simulink model "grid_tied_Inverter"  (R2013a)
settings: Solver=ode45  SolverMode=SingleTasking  StartTime=0.0  StopTime=5  FixedStep=0.00001  RelTol=1e-3
libraries: powerlib x15, simulink_extras x2, powerlib_extras x2, simulink x1
settings Model: Creator=lang  LastModifiedBy=Yooshaa
settings DataIOCC: SignalLoggingSaveFormat=ModelDataLogs
settings OptimizationCC: BlockReduction=off  BooleanDataType=off  InlineParams=on
settings DebuggingCC: SaveWithParameterizedLinksMsg=none  SignalResolutionControl=TryResolveAllWithWarning  SolverPrmCheckMsg=none  MultiTaskDSMMsg=warning  MultiTaskCondExecSysMsg=none  StrictBusMsg=None
settings HardwareCC: TargetUnknown=on
settings RTWCC: IncludeERTFirstTime=on

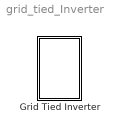
== system grid_tied_Inverter ==
  Grid Tied Inverter : Subsystem  mask{Vdc=1200, Pb=2.3e6, Vp=((690*(2^0.5))/(3^0.5)), Fb=60, Vbase=((690*(2^0.5))/(3^0.5))/(2^.5), Ibase=(2.3e6/3)/(690/(3^0.5)), Grid_Angle_init=pi, Lgrid=0.1098e-3, Fs=1e4, Fsampling=2e4, Kp=1, Ki=2, P_desired_pu=3, Q_desired_pu=0}

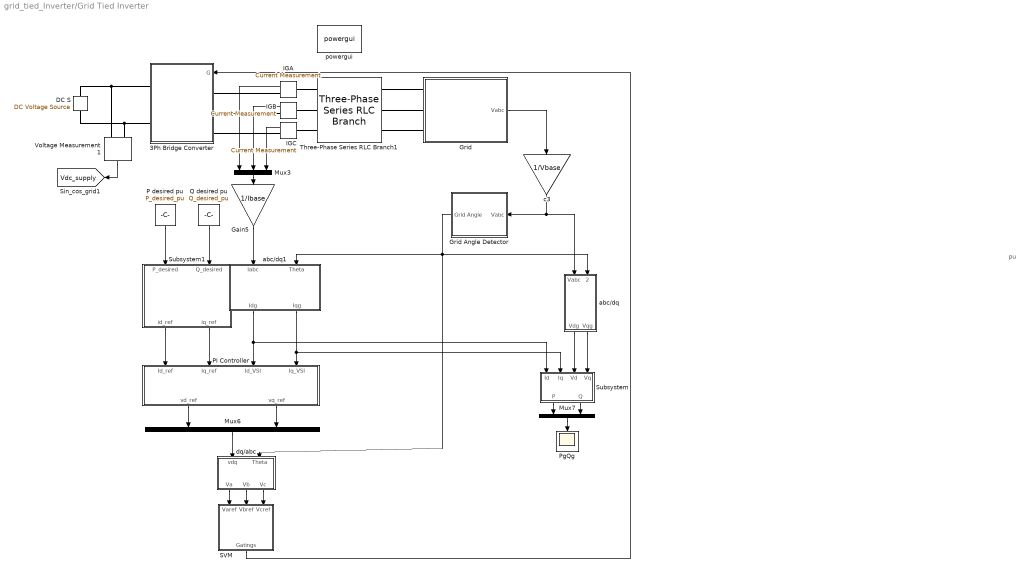
== system grid_tied_Inverter/Grid Tied Inverter ==
  note: pu
  3Ph Bridge Converter : Subsystem
  DC S : powerlib/Electrical Sources/DC Voltage Source  Amplitude=Vdc  Measurements=None
  Gain5 : Gain  Gain=1/Ibase
  Grid : Subsystem
  Grid Angle Detector : Subsystem
  IGA : powerlib/Measurements/Current Measurement  PhasorSimulation=off  OutputType=Complex  PSBequivalent=0
  IGB : powerlib/Measurements/Current Measurement  PhasorSimulation=off  OutputType=Complex  PSBequivalent=0
  IGC : powerlib/Measurements/Current Measurement  PhasorSimulation=off  OutputType=Complex  PSBequivalent=0
  Mux3 : Mux  Inputs=3
  Mux6 : Mux  Inputs=2
  Mux7 : Mux  Inputs=2
  P desired pu : Constant  Value=P_desired_pu
  PI Controller : Subsystem
  PgQg : Scope
      settings: YMin=-2  YMax=6  SaveName=ScopeData7
  Q desired pu : Constant  Value=Q_desired_pu
  SVM : Subsystem
  Subsystem : Subsystem
  Subsystem1 : Subsystem
  Three-Phase Series RLC Branch1 : powerlib/Elements/Three-Phase Series RLC Branch  LConnTagsString=A|B|C  RConnTagsString=A|B|C  BranchType=L  Resistance=1e-6  Inductance=Lgrid  Capacitance=1e-6  Measurements=Branch currents
  Voltage Measurement1 : powerlib/Measurements/Voltage Measurement  PhasorSimulation=off  OutputType=Complex  PSBequivalent=0
  abc/dq : Subsystem
  abc/dq1 : Subsystem
  c3 : Gain  Gain=1/Vbase
  dq/abc : Subsystem
  powergui : powerlib/powergui  Priority=1  SimulationMode=Continuous  SolverType=Tustin  SampleTime=50e-6  frequency=60  SPID=on  DisableSnubberDevices=off  DisableRonSwitches=off  DisableVfSwitches=off  SwTol=0  Interpol=off  DisplayEquations=off  frequencyindice=0  Pbase=100e6  ErrMax=1e-4  Iterations=50  UnitsV=kV  UnitsW=MW  FunctionMessages=off  echomessages=off  HookPort=off  EnableUseOfTLC=off  x0status=blocks  RestoreLinks=warning  ResistiveCurrentMeasurement=off  Frange=[0:2:500]  Ylog=off  Xlog=on  ShowGrid=off  save=off  variable=ZData  ZoomFFT=off  StartTime=0.0  cycles=1  DisplayStyle=1  fundamental=60  FreqAxis=off  MaxFrequency=1000  frequencyindicesteady=1  RmsSteady=1  display=off  Ts=0  methode=off
  tag scope: Vdc_supply=global
  wires:
  Voltage Measurement1/1 -> [Vdc_supply]
  SVM/1(Gatings) -> 3Ph Bridge Converter/1(G)
  dq/abc/2(Vb) -> SVM/2(Vbref)
  Grid/1(Vabc) -> c3/1
  dq/abc/3(Vc) -> SVM/3(Vcref)
  dq/abc/1(Va) -> SVM/1(Varef)
  abc/dq/1(Vdg) -> Subsystem/3(Vd)
  Subsystem1/1(id_ref) -> PI Controller/1(Id_ref)
  abc/dq1/1(Idg) -> PI Controller/3(Id_VSI), Subsystem/1(Id)
  Mux3/1 -> Gain5/1
  PI Controller/2(vq_ref) -> Mux6/2
  IGC/1 -> Mux3/3
  c3/1 -> Grid Angle Detector/1(Vabc), abc/dq/1(Vabc)
  Mux6/1 -> dq/abc/1(vdq)
  Mux7/1 -> PgQg/1
  Subsystem1/2(iq_ref) -> PI Controller/2(Iq_ref)
  Subsystem/2(Q) -> Mux7/2
  IGA/1 -> Mux3/1
  Gain5/1 -> abc/dq1/1(Iabc)
  Subsystem/1(P) -> Mux7/1
  abc/dq1/2(Iqg) -> Subsystem/2(Iq), PI Controller/4(Iq_VSI)
  IGB/1 -> Mux3/2
  Grid Angle Detector/1(Grid Angle) -> dq/abc/2(Theta), abc/dq1/2(Theta), abc/dq/2(Theta)
  PI Controller/1(vd_ref) -> Mux6/1
  abc/dq/2(Vqg) -> Subsystem/4(Vq)
  P desired pu/1 -> Subsystem1/1(P_desired)
  Q desired pu/1 -> Subsystem1/2(Q_desired)
  connections:
  3Ph Bridge Converter/RConn1 -- DC S/RConn1 -- Voltage Measurement1/LConn1
  3Ph Bridge Converter/RConn2 -- DC S/LConn1 -- Voltage Measurement1/LConn2
  IGC/RConn1 -- 3Ph Bridge Converter/LConn3
  Three-Phase Series RLC Branch1/RConn1 -- IGA/LConn1
  Three-Phase Series RLC Branch1/RConn3 -- IGC/LConn1
  3Ph Bridge Converter/LConn1 -- IGA/RConn1
  Three-Phase Series RLC Branch1/RConn2 -- IGB/LConn1
  Grid/LConn1 -- Three-Phase Series RLC Branch1/LConn1
  Grid/LConn2 -- Three-Phase Series RLC Branch1/LConn2
  3Ph Bridge Converter/LConn2 -- IGB/RConn1
  Grid/LConn3 -- Three-Phase Series RLC Branch1/LConn3

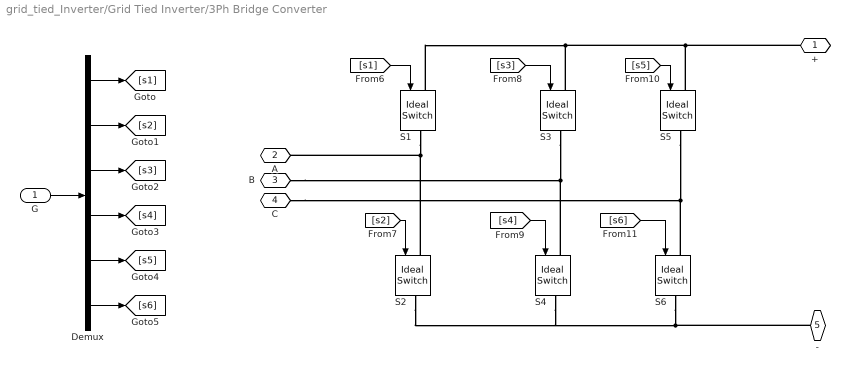
== system grid_tied_Inverter/Grid Tied Inverter/3Ph Bridge Converter ==
  G : Inport
   S{1..6} (6 alike) : powerlib/Power Electronics/Ideal Switch  Ron=0  Lon=0  IC=0  Rs=inf  Cs=inf  Measurements=off
  Demux : Demux  Outputs=6
  + : PMIOPort  Port=1  Side=Right
  A : PMIOPort  Port=2  Side=Left
  B : PMIOPort  Port=3  Side=Left
  C : PMIOPort  Port=4  Side=Left
  - : PMIOPort  Port=5  Side=Right
  wires:
  [s1] -> " S1"/1
  [s5] -> " S5"/1
  Demux/1 -> [s1]
  Demux/2 -> [s2]
  Demux/3 -> [s3]
  Demux/4 -> [s4]
  Demux/5 -> [s5]
  Demux/6 -> [s6]
  G/1 -> Demux/1
  [s2] -> " S2"/1
  [s3] -> " S3"/1
  [s4] -> " S4"/1
  [s6] -> " S6"/1
  connections:
  +/RConn1 -- " S1"/LConn1 -- " S3"/LConn1 -- " S5"/LConn1
  -/RConn1 -- " S2"/RConn1 -- " S4"/RConn1 -- " S6"/RConn1
  " S1"/RConn1 -- " S2"/LConn1 -- A/RConn1
  B/RConn1 -- " S4"/LConn1 -- " S3"/RConn1
  C/RConn1 -- " S6"/LConn1 -- " S5"/RConn1

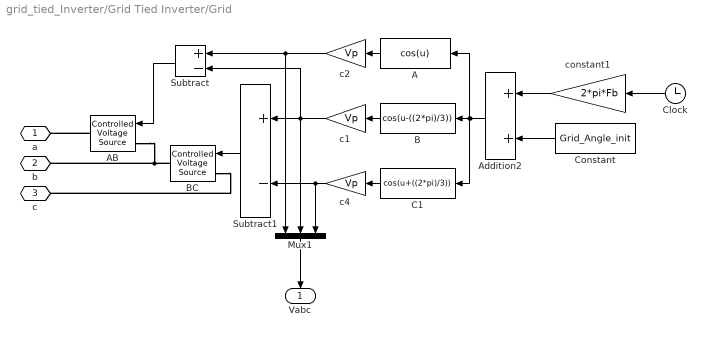
== system grid_tied_Inverter/Grid Tied Inverter/Grid ==
  A : Fcn  Expr=cos(u)
  AB : powerlib/Electrical Sources/Controlled Voltage Source  Initialize=off  Source_Type=AC  Amplitude=0  Phase=0  Frequency=0  Measurements=None
  Addition2 : Sum
  B : Fcn  Expr=cos(u-((2*pi)/3))
  BC : powerlib/Electrical Sources/Controlled Voltage Source  Initialize=off  Source_Type=AC  Amplitude=0  Phase=0  Frequency=0  Measurements=None
  C1 : Fcn  Expr=cos(u+((2*pi)/3))
  Clock : Clock
  Constant : Constant  Value=Grid_Angle_init
  Mux1 : Mux  Inputs=3
  Subtract : Sum  Inputs=+-
  Subtract1 : Sum  Inputs=+-
  c1 : Gain  Gain=Vp
  c2 : Gain  Gain=Vp
  c4 : Gain  Gain=Vp
  constant1 : Gain  Gain=2*pi*Fb
  a : PMIOPort  Port=1  Side=Left
  b : PMIOPort  Port=2  Side=Left
  c : PMIOPort  Port=3  Side=Left
  Vabc : Outport
  wires:
  c4/1 -> Subtract1/2, Mux1/3
  constant1/1 -> Addition2/1
  c1/1 -> Subtract1/1, Mux1/2, Subtract/2
  Addition2/1 -> C1/1, A/1, B/1
  Constant/1 -> Addition2/2
  B/1 -> c1/1
  C1/1 -> c4/1
  Clock/1 -> constant1/1
  c2/1 -> Subtract/1, Mux1/1
  A/1 -> c2/1
  Subtract1/1 -> BC/1
  Mux1/1 -> Vabc/1
  Subtract/1 -> AB/1
  connections:
  AB/RConn1 -- a/RConn1
  BC/RConn1 -- b/RConn1 -- AB/LConn1
  BC/LConn1 -- c/RConn1

== system grid_tied_Inverter/Grid Tied Inverter/Grid Angle Detector ==
  Vabc : Inport
  Add : Sum
  Beta1 : Fcn  Expr=(1/(3^.5))*(u(1)+2*u(2))
  Cartesian to Polar1 : simulink_extras/Transformations/Cartesian to Polar
  Constant : Constant  Value=2*pi
  Math Function : Math  Operator=rem  SaturateOnIntegerOverflow=on
  Unit Delay3 : UnitDelay  InitialCondition=Grid_Angle_init  SampleTime=1/Fsampling
  alpha1 : Fcn  Expr=u(1)
  Grid Angle : Outport
  wires:
  Beta1/1 -> Cartesian to Polar1/2
  Vabc/1 -> alpha1/1, Beta1/1
  Unit Delay3/1 -> Grid Angle/1
  alpha1/1 -> Cartesian to Polar1/1
  Cartesian to Polar1/2 -> Add/1
  Constant/1 -> Math Function/2, Add/2
  Add/1 -> Math Function/1
  Math Function/1 -> Unit Delay3/1

== system grid_tied_Inverter/Grid Tied Inverter/PI Controller ==
  Id_ref : Inport
  Iq_ref : Inport  Port=2
  Id_VSI : Inport  Port=3
  Iq_VSI : Inport  Port=4
  Sum : Sum  Inputs=|-+
  Sum2 : Sum  Inputs=|-+
  id_Ctr1 : powerlib_extras/Discrete  Control Blocks/Discrete PI Controller  Kp=Kp  Ki=Ki  Par_Limits=[1e6 -1e6]  Init=0  Ts=50e-6
  iq_Ctr2 : powerlib_extras/Discrete  Control Blocks/Discrete PI Controller  Kp=Kp  Ki=Ki  Par_Limits=[1e6 -1e6]  Init=0  Ts=50e-6
  vd_ref : Outport
  vq_ref : Outport  Port=2
  wires:
  Iq_VSI/1 -> Sum2/2
  Sum/1 -> id_Ctr1/1
  Sum2/1 -> iq_Ctr2/1
  Id_ref/1 -> Sum/1
  Iq_ref/1 -> Sum2/1
  iq_Ctr2/1 -> vq_ref/1
  id_Ctr1/1 -> vd_ref/1
  Id_VSI/1 -> Sum/2

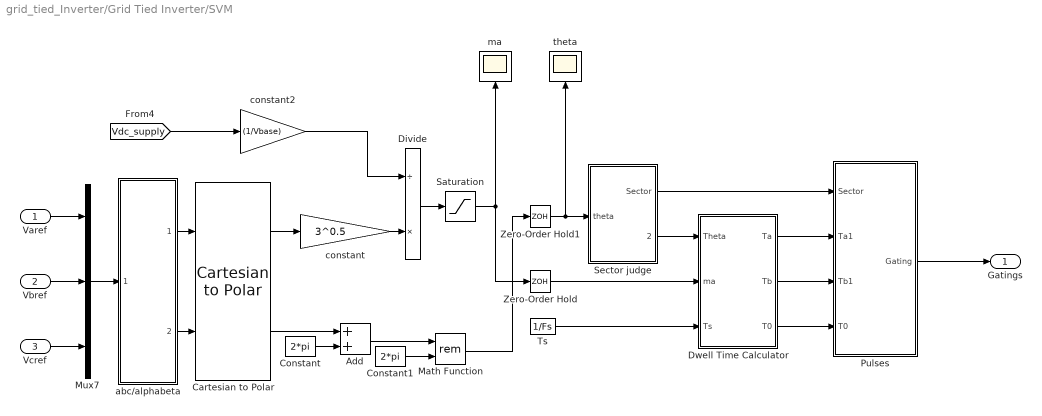
== system grid_tied_Inverter/Grid Tied Inverter/SVM ==
  Varef : Inport
  Vbref : Inport  Port=2
  Vcref : Inport  Port=3
  Add : Sum
  Cartesian to Polar : simulink_extras/Transformations/Cartesian to Polar
  Constant : Constant  Value=2*pi
  Constant1 : Constant  Value=2*pi
  Divide : Product  Inputs=/*
  Dwell Time Calculator : Subsystem
  Math Function : Math  Operator=rem  SaturateOnIntegerOverflow=on
  Mux7 : Mux  Inputs=3
  Pulses : Subsystem
  Saturation : Saturate  UpperLimit=1  LowerLimit=0  SampleTime=1/Fsampling
  Sector judge : Subsystem
  Ts : Constant  Value=1/Fs
  Zero-Order Hold : ZeroOrderHold  SampleTime=1/(2*Fs)
  Zero-Order Hold1 : ZeroOrderHold  SampleTime=1/(2*Fs)
  abc/alphabeta : Subsystem
  constant : Gain  Gain=3^0.5
  constant2 : Gain  Gain=(1/Vbase)
  ma : Scope
      settings: SaveName=ScopeData5
  theta : Scope
      settings: YMin=0  YMax=6.5  SaveName=ScopeData6
  Gatings : Outport
  wires:
  Dwell Time Calculator/3(T0) -> Pulses/4(T0)
  constant/1 -> Divide/2
  Pulses/1(Gating) -> Gatings/1
  Cartesian to Polar/1 -> constant/1
  Divide/1 -> Saturation/1
  Ts/1 -> Dwell Time Calculator/3(Ts)
  Varef/1 -> Mux7/1
  Dwell Time Calculator/1(Ta) -> Pulses/2(Ta1)
  Dwell Time Calculator/2(Tb) -> Pulses/3(Tb1)
  Sector judge/2(Cal_theta) -> Dwell Time Calculator/1(Theta)
  Saturation/1 -> Zero-Order Hold/1, ma/1
  Zero-Order Hold/1 -> Dwell Time Calculator/2(ma)
  constant2/1 -> Divide/1
  Zero-Order Hold1/1 -> Sector judge/1(theta), theta/1
  Sector judge/1(Sector) -> Pulses/1(Sector)
  abc/alphabeta/1(Valpha) -> Cartesian to Polar/1
  Mux7/1 -> abc/alphabeta/1(Vabc)
  Vbref/1 -> Mux7/2
  abc/alphabeta/2(Vbeta) -> Cartesian to Polar/2
  Vcref/1 -> Mux7/3
  Cartesian to Polar/2 -> Add/1
  Math Function/1 -> Zero-Order Hold1/1
  Constant/1 -> Add/2
  Add/1 -> Math Function/1
  Constant1/1 -> Math Function/2
  [Vdc_supply] -> constant2/1

== system grid_tied_Inverter/Grid Tied Inverter/Subsystem ==
  Id : Inport
  Iq : Inport  Port=2
  Vd : Inport  Port=3
  Vq : Inport  Port=4
  Add : Sum
  Add1 : Sum  Inputs=+-
  Gain : Gain  Gain=3/2
  Gain1 : Gain  Gain=3/2
  Product{,1..3} (4 alike) : Product
  Scope : Scope  NumInputPorts=4
      settings: YMin=0.5~-1~1.41~0.05  YMax=2.75~1~1.41325~0.11
  P : Outport
  Q : Outport  Port=2
  tag scope: vd=global, vq=global
  wires:
  Id/1 -> Scope/1, Product2/1, Product/1
  Vd/1 -> [vd], Scope/3, Product3/2, Product/2
  Iq/1 -> Scope/2, Product3/1, Product1/1
  Vq/1 -> [vq], Scope/4, Product2/2, Product1/2
  Product/1 -> Add/1
  Product1/1 -> Add/2
  Add/1 -> Gain/1
  Gain/1 -> P/1
  Product2/1 -> Add1/1
  Product3/1 -> Add1/2
  Add1/1 -> Gain1/1
  Gain1/1 -> Q/1

== system grid_tied_Inverter/Grid Tied Inverter/Subsystem1 ==
  P_desired : Inport
  Q_desired : Inport  Port=2
  Fcn : Fcn  Expr=((-2/3)*(u(3)*u(2)-u(4)*u(1)))/(u(3)*u(3)+u(4)*u(4))
  Fcn1 : Fcn  Expr=((2*u(1)/3)-u(4)*(((-2/3)*(u(3)*u(2)-u(4)*u(1)))/(u(3)*u(3)+u(4)*u(4))))/u(3)
  Mux : Mux
  Scope : Scope  NumInputPorts=2
      settings: YMin=-2~-2  YMax=2~2  SaveName=ScopeData3
  id_ref : Outport
  iq_ref : Outport  Port=2
  wires:
  [vq] -> Mux/4
  [vd] -> Mux/3
  Q_desired/1 -> Mux/2
  P_desired/1 -> Mux/1
  Mux/1 -> Fcn1/1, Fcn/1
  Fcn1/1 -> Scope/2, id_ref/1
  Fcn/1 -> Scope/1, iq_ref/1

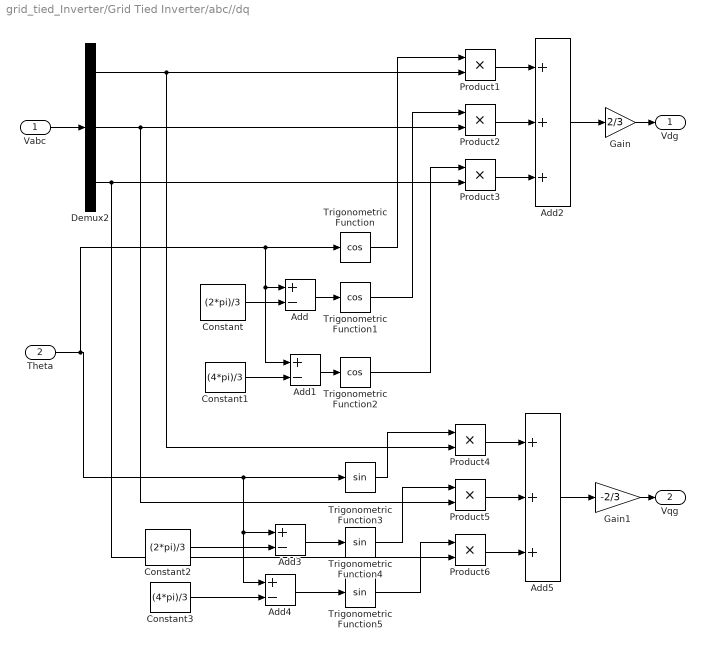
== system grid_tied_Inverter/Grid Tied Inverter/abc//dq ==
  Vabc : Inport
  Theta : Inport  Port=2
  Add{,1,3..4} (4 alike) : Sum  Inputs=+-
  Add2 : Sum  Inputs=+++
  Add5 : Sum  Inputs=+++
  Constant : Constant  Value=(2*pi)/3
  Constant1 : Constant  Value=(4*pi)/3
  Constant2 : Constant  Value=(2*pi)/3
  Constant3 : Constant  Value=(4*pi)/3
  Demux2 : Demux  Outputs=3
  Gain : Gain  Gain=2/3
  Gain1 : Gain  Gain=-2/3
  Product{1..6} (6 alike) : Product
  Trigonometric Function : Trigonometry  Operator=cos
  Trigonometric Function1 : Trigonometry  Operator=cos
  Trigonometric Function2 : Trigonometry  Operator=cos
  Trigonometric Function3 : Trigonometry
  Trigonometric Function4 : Trigonometry
  Trigonometric Function5 : Trigonometry
  Vdg : Outport
  Vqg : Outport  Port=2
  wires:
  Trigonometric Function1/1 -> Product2/1
  Constant/1 -> Add/2
  Trigonometric Function/1 -> Product1/1
  Trigonometric Function2/1 -> Product3/1
  Add/1 -> Trigonometric Function1/1
  Constant1/1 -> Add1/2
  Product2/1 -> Add2/2
  Product1/1 -> Add2/1
  Constant2/1 -> Add3/2
  Demux2/1 -> Product4/2, Product1/2
  Product5/1 -> Add5/2
  Constant3/1 -> Add4/2
  Add4/1 -> Trigonometric Function5/1
  Trigonometric Function3/1 -> Product4/1
  Trigonometric Function4/1 -> Product5/1
  Add3/1 -> Trigonometric Function4/1
  Trigonometric Function5/1 -> Product6/1
  Demux2/2 -> Product5/2, Product2/2
  Demux2/3 -> Product6/2, Product3/2
  Product4/1 -> Add5/1
  Add5/1 -> Gain1/1
  Product6/1 -> Add5/3
  Add1/1 -> Trigonometric Function2/1
  Product3/1 -> Add2/3
  Theta/1 -> Trigonometric Function/1, Add1/1, Add/1, Add4/1, Add3/1, Trigonometric Function3/1
  Vabc/1 -> Demux2/1
  Gain/1 -> Vdg/1
  Add2/1 -> Gain/1
  Gain1/1 -> Vqg/1

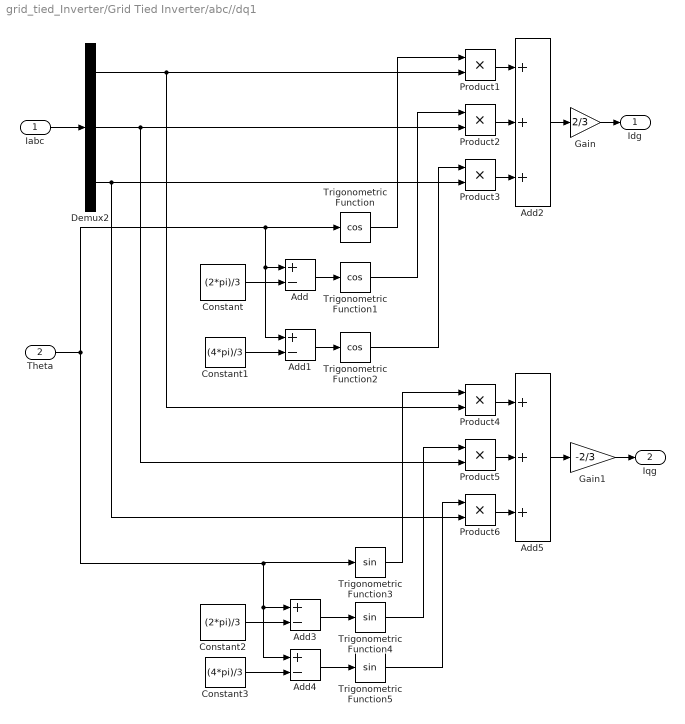
== system grid_tied_Inverter/Grid Tied Inverter/abc//dq1 ==
  Iabc : Inport
  Theta : Inport  Port=2
  Add{,1,3..4} (4 alike) : Sum  Inputs=+-
  Add2 : Sum  Inputs=+++
  Add5 : Sum  Inputs=+++
  Constant : Constant  Value=(2*pi)/3
  Constant1 : Constant  Value=(4*pi)/3
  Constant2 : Constant  Value=(2*pi)/3
  Constant3 : Constant  Value=(4*pi)/3
  Demux2 : Demux  Outputs=3
  Gain : Gain  Gain=2/3
  Gain1 : Gain  Gain=-2/3
  Product{1..6} (6 alike) : Product
  Trigonometric Function : Trigonometry  Operator=cos
  Trigonometric Function1 : Trigonometry  Operator=cos
  Trigonometric Function2 : Trigonometry  Operator=cos
  Trigonometric Function3 : Trigonometry
  Trigonometric Function4 : Trigonometry
  Trigonometric Function5 : Trigonometry
  Idg : Outport
  Iqg : Outport  Port=2
  wires:
  Trigonometric Function1/1 -> Product2/1
  Constant/1 -> Add/2
  Trigonometric Function/1 -> Product1/1
  Trigonometric Function2/1 -> Product3/1
  Add/1 -> Trigonometric Function1/1
  Constant1/1 -> Add1/2
  Product2/1 -> Add2/2
  Product1/1 -> Add2/1
  Constant2/1 -> Add3/2
  Demux2/1 -> Product4/2, Product1/2
  Product5/1 -> Add5/2
  Constant3/1 -> Add4/2
  Add4/1 -> Trigonometric Function5/1
  Trigonometric Function3/1 -> Product4/1
  Trigonometric Function4/1 -> Product5/1
  Add3/1 -> Trigonometric Function4/1
  Trigonometric Function5/1 -> Product6/1
  Demux2/2 -> Product5/2, Product2/2
  Demux2/3 -> Product6/2, Product3/2
  Product4/1 -> Add5/1
  Add5/1 -> Gain1/1
  Product6/1 -> Add5/3
  Add1/1 -> Trigonometric Function2/1
  Product3/1 -> Add2/3
  Theta/1 -> Trigonometric Function/1, Add1/1, Add/1, Add4/1, Add3/1, Trigonometric Function3/1
  Gain1/1 -> Iqg/1
  Iabc/1 -> Demux2/1
  Gain/1 -> Idg/1
  Add2/1 -> Gain/1

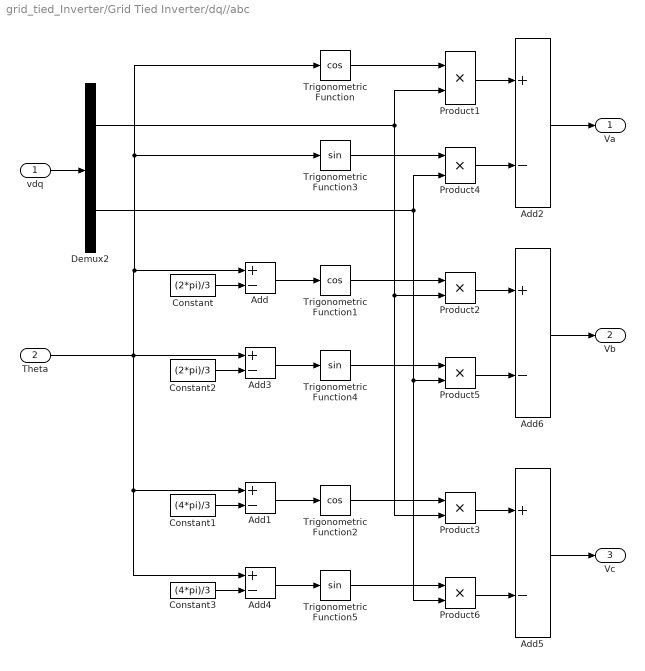
== system grid_tied_Inverter/Grid Tied Inverter/dq//abc ==
  vdq : Inport
  Theta : Inport  Port=2
  Add{,1..6} (7 alike) : Sum  Inputs=+-
  Constant : Constant  Value=(2*pi)/3
  Constant1 : Constant  Value=(4*pi)/3
  Constant2 : Constant  Value=(2*pi)/3
  Constant3 : Constant  Value=(4*pi)/3
  Demux2 : Demux  Outputs=2
  Product{1..6} (6 alike) : Product
  Trigonometric Function : Trigonometry  Operator=cos
  Trigonometric Function1 : Trigonometry  Operator=cos
  Trigonometric Function2 : Trigonometry  Operator=cos
  Trigonometric Function3 : Trigonometry
  Trigonometric Function4 : Trigonometry
  Trigonometric Function5 : Trigonometry
  Va : Outport
  Vb : Outport  Port=2
  Vc : Outport  Port=3
  wires:
  Trigonometric Function1/1 -> Product2/1
  Constant/1 -> Add/2
  Trigonometric Function/1 -> Product1/1
  Add/1 -> Trigonometric Function1/1
  Product1/1 -> Add2/1
  Constant2/1 -> Add3/2
  Demux2/1 -> Product1/2, Product2/2, Product3/2
  Trigonometric Function3/1 -> Product4/1
  Trigonometric Function4/1 -> Product5/1
  Add3/1 -> Trigonometric Function4/1
  vdq/1 -> Demux2/1
  Add2/1 -> Va/1
  Product4/1 -> Add2/2
  Demux2/2 -> Product4/2, Product6/2, Product5/2
  Product2/1 -> Add6/1
  Add6/1 -> Vb/1
  Product5/1 -> Add6/2
  Trigonometric Function2/1 -> Product3/1
  Constant1/1 -> Add1/2
  Add1/1 -> Trigonometric Function2/1
  Constant3/1 -> Add4/2
  Trigonometric Function5/1 -> Product6/1
  Add4/1 -> Trigonometric Function5/1
  Theta/1 -> Trigonometric Function/1, Trigonometric Function3/1, Add/1, Add4/1, Add1/1, Add3/1
  Product3/1 -> Add5/1
  Add5/1 -> Vc/1
  Product6/1 -> Add5/2

== system grid_tied_Inverter/Grid Tied Inverter/SVM/Dwell Time Calculator ==
  Theta : Inport
  ma : Inport  Port=2
  Ts : Inport  Port=3
  Add : Sum  Inputs=--+
  Compare To Zero : simulink/Logic and Bit Operations/Compare To Zero  relop=>=  OutDataTypeStr=boolean
  Data Type Conversion : DataTypeConversion  OutDataTypeStr=double
  Mux : Mux  Inputs=3
  Product : Product  RndMeth=Zero
  Scope : Scope  NumInputPorts=3
      settings: YMin=1.25e-05~0~0  YMax=4.25e-05~8.5e-05~8.5e-05  SaveName=ScopeData12
  cTa : Fcn  Expr=u(2)*u(3)*sin((pi/3)-u(1))
  cTb : Fcn  Expr=u(2)*u(3)*sin(u(1))
  Ta : Outport
  Tb : Outport  Port=2
  T0 : Outport  Port=3
  wires:
  Product/1 -> Scope/1, T0/1
  Theta/1 -> Mux/1
  ma/1 -> Mux/2
  Ts/1 -> Add/3, Mux/3
  Mux/1 -> cTb/1, cTa/1
  Add/1 -> Product/2, Compare To Zero/1
  Data Type Conversion/1 -> Product/1
  Compare To Zero/1 -> Data Type Conversion/1
  cTa/1 -> Scope/2, Ta/1, Add/1
  cTb/1 -> Scope/3, Tb/1, Add/2

== system grid_tied_Inverter/Grid Tied Inverter/SVM/Pulses ==
  Sector : Inport
  Ta1 : Inport  Port=2
  Tb1 : Inport  Port=3
  T0 : Inport  Port=4
  Inverter Leg a : Subsystem
  Inverter Leg b : Subsystem
  Inverter Leg c : Subsystem
  Logical Operator : Logic  Operator=NOT  AllPortsSameDT=off
  Logical Operator1 : Logic  Operator=NOT  AllPortsSameDT=off
  Logical Operator2 : Logic  Operator=NOT  AllPortsSameDT=off
  Mux : Mux  Inputs=6
  Scope1 : Scope
      settings: SaveName=ScopeData2
  Sector Select a : MultiPortSwitch  Inputs=6
  Sector Select b : MultiPortSwitch  Inputs=6
  Sector Select c : MultiPortSwitch  Inputs=6
  Switching Segment Calculator : Subsystem
  Gating : Outport
  wires:
  Sector/1 -> Sector Select a/1, Scope1/1, Sector Select b/1, Sector Select c/1
  Sector Select a/1 -> Logical Operator/1, Mux/1
  Sector Select b/1 -> Logical Operator1/1, Mux/3
  Sector Select c/1 -> Logical Operator2/1, Mux/5
  Mux/1 -> Gating/1
  Logical Operator/1 -> Mux/2
  Logical Operator1/1 -> Mux/4
  Logical Operator2/1 -> Mux/6
  Switching Segment Calculator/1(Segment) -> Inverter Leg c/1(Segment), Inverter Leg a/1(Segment), Inverter Leg b/1(Segment)
  T0/1 -> Switching Segment Calculator/1(T0)
  Ta1/1 -> Switching Segment Calculator/2(Ta)
  Tb1/1 -> Switching Segment Calculator/3(Tb)
  Inverter Leg a/1(Out1) -> Sector Select a/2
  Inverter Leg a/2(Out2) -> Sector Select a/3
  Inverter Leg a/3(Out3) -> Sector Select a/4
  Inverter Leg a/4(Out4) -> Sector Select a/5
  Inverter Leg a/5(Out5) -> Sector Select a/6
  Inverter Leg a/6(Out6) -> Sector Select a/7
  Inverter Leg b/1(Out1) -> Sector Select b/2
  Inverter Leg b/2(Out2) -> Sector Select b/3
  Inverter Leg b/3(Out3) -> Sector Select b/4
  Inverter Leg b/4(Out4) -> Sector Select b/5
  Inverter Leg b/5(Out5) -> Sector Select b/6
  Inverter Leg b/6(Out6) -> Sector Select b/7
  Inverter Leg c/1(Out1) -> Sector Select c/2
  Inverter Leg c/2(Out2) -> Sector Select c/3
  Inverter Leg c/3(Out3) -> Sector Select c/4
  Inverter Leg c/4(Out4) -> Sector Select c/5
  Inverter Leg c/5(Out5) -> Sector Select c/6
  Inverter Leg c/6(Out6) -> Sector Select c/7

== system grid_tied_Inverter/Grid Tied Inverter/SVM/Sector judge ==
  theta : Inport
  Add : Sum
  Constant : Constant  Value=2*pi
  Constant1 : Constant  OutDataTypeStr=boolean
  Constant2 : Constant  Value=2*pi
  Gain1 : Gain  Gain=3/pi
  Gain2 : Gain  Gain=pi/3
  Math Function1 : Math  Operator=rem  SaturateOnIntegerOverflow=on
  Rounding Function : Rounding
  Sum1 : Sum  Inputs=|++  SaturateOnIntegerOverflow=on
  Sum2 : Sum  Inputs=|-+
  Sector : Outport
  Cal_theta : Outport  Port=2
  wires:
  Gain1/1 -> Rounding Function/1
  Rounding Function/1 -> Gain2/1, Sum1/1
  Sum1/1 -> Sector/1
  Constant1/1 -> Sum1/2
  Gain2/1 -> Sum2/1
  Sum2/1 -> Cal_theta/1
  theta/1 -> Add/1
  Math Function1/1 -> Sum2/2, Gain1/1
  Constant/1 -> Add/2
  Add/1 -> Math Function1/1
  Constant2/1 -> Math Function1/2

== system grid_tied_Inverter/Grid Tied Inverter/SVM/abc//alphabeta ==
  Vabc : Inport
  Beta1 : Fcn  Expr=(1/(3^.5))*(u(1)+2*u(2))
  alpha1 : Fcn  Expr=u(1)
  Valpha : Outport
  Vbeta : Outport  Port=2
  wires:
  Vabc/1 -> Beta1/1, alpha1/1
  alpha1/1 -> Valpha/1
  Beta1/1 -> Vbeta/1

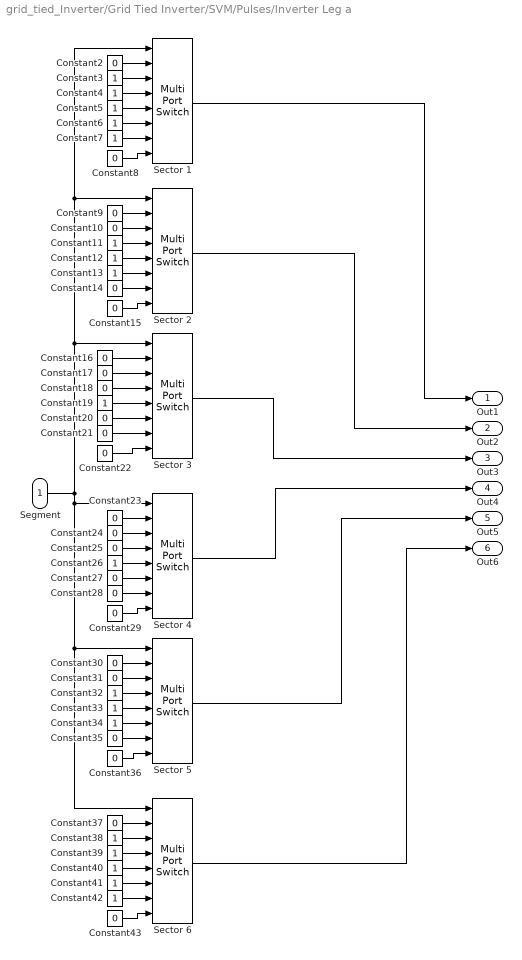
== system grid_tied_Inverter/Grid Tied Inverter/SVM/Pulses/Inverter Leg a ==
  Segment : Inport
  Constant{2,8..10,14..18,20..25,27..31,35..37,43} (24 alike) : Constant  Value=0
  Constant{3..7,11..13,19,26,32..34,38..42} (18 alike) : Constant
  Sector {1..6} (6 alike) : MultiPortSwitch  Inputs=7
  Out1 : Outport
  Out2 : Outport  Port=2
  Out3 : Outport  Port=3
  Out4 : Outport  Port=4
  Out5 : Outport  Port=5
  Out6 : Outport  Port=6
  wires:
  Segment/1 -> Sector 6/1, Sector 5/1, Sector 4/1, Sector 2/1, Sector 1/1, Sector 3/1
  Sector 3/1 -> Out3/1
  Constant2/1 -> Sector 1/2
  Constant7/1 -> Sector 1/7
  Sector 1/1 -> Out1/1
  Constant3/1 -> Sector 1/3
  Constant6/1 -> Sector 1/6
  Constant10/1 -> Sector 2/3
  Sector 6/1 -> Out6/1
  Sector 2/1 -> Out2/1
  Constant5/1 -> Sector 1/5
  Constant9/1 -> Sector 2/2
  Constant4/1 -> Sector 1/4
  Constant8/1 -> Sector 1/8
  Sector 4/1 -> Out4/1
  Sector 5/1 -> Out5/1
  Constant42/1 -> Sector 6/7
  Constant43/1 -> Sector 6/8
  Constant40/1 -> Sector 6/5
  Constant37/1 -> Sector 6/2
  Constant41/1 -> Sector 6/6
  Constant39/1 -> Sector 6/4
  Constant17/1 -> Sector 3/3
  Constant30/1 -> Sector 5/2
  Constant38/1 -> Sector 6/3
  Constant29/1 -> Sector 4/8
  Constant28/1 -> Sector 4/7
  Constant31/1 -> Sector 5/3
  Constant25/1 -> Sector 4/4
  Constant20/1 -> Sector 3/6
  Constant26/1 -> Sector 4/5
  Constant32/1 -> Sector 5/4
  Constant33/1 -> Sector 5/5
  Constant36/1 -> Sector 5/8
  Constant18/1 -> Sector 3/4
  Constant14/1 -> Sector 2/7
  Constant13/1 -> Sector 2/6
  Constant34/1 -> Sector 5/6
  Constant24/1 -> Sector 4/3
  Constant11/1 -> Sector 2/4
  Constant16/1 -> Sector 3/2
  Constant21/1 -> Sector 3/7
  Constant12/1 -> Sector 2/5
  Constant19/1 -> Sector 3/5
  Constant35/1 -> Sector 5/7
  Constant22/1 -> Sector 3/8
  Constant23/1 -> Sector 4/2
  Constant15/1 -> Sector 2/8
  Constant27/1 -> Sector 4/6

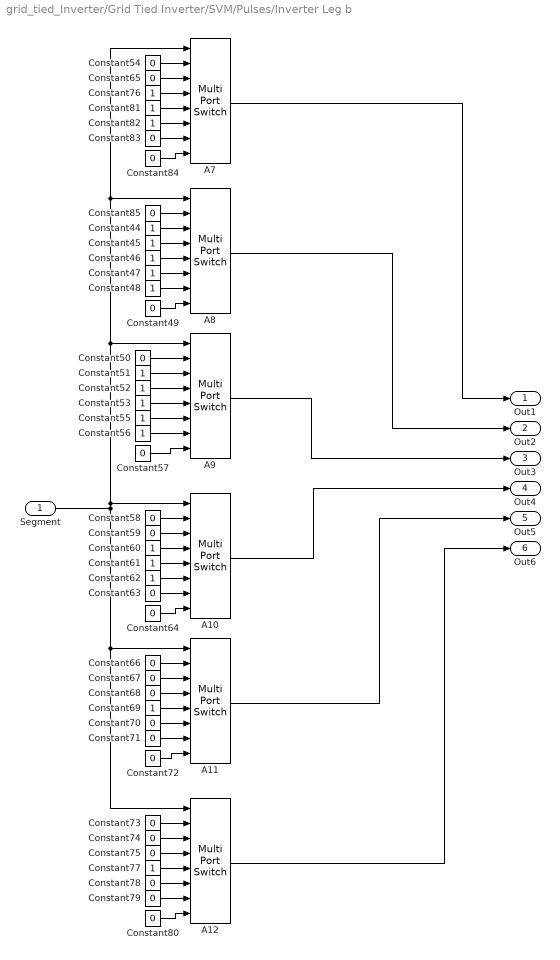
== system grid_tied_Inverter/Grid Tied Inverter/SVM/Pulses/Inverter Leg b ==
  Segment : Inport
  A{7..12} (6 alike) : MultiPortSwitch  Inputs=7
  Constant{44..48,51..53,55..56,60..62,69,76..77,81..82} (18 alike) : Constant
  Constant{49..50,54,57..59,63..68,70..75,78..80,83..85} (24 alike) : Constant  Value=0
  Out1 : Outport
  Out2 : Outport  Port=2
  Out3 : Outport  Port=3
  Out4 : Outport  Port=4
  Out5 : Outport  Port=5
  Out6 : Outport  Port=6
  wires:
  Segment/1 -> A7/1, A8/1, A9/1, A10/1, A12/1, A11/1
  Constant80/1 -> A12/8
  Constant71/1 -> A11/7
  Constant69/1 -> A11/5
  Constant70/1 -> A11/6
  Constant72/1 -> A11/8
  Constant73/1 -> A12/2
  Constant75/1 -> A12/4
  Constant77/1 -> A12/5
  Constant79/1 -> A12/7
  Constant74/1 -> A12/3
  Constant68/1 -> A11/4
  Constant78/1 -> A12/6
  Constant55/1 -> A9/6
  Constant61/1 -> A10/5
  Constant47/1 -> A8/6
  Constant53/1 -> A9/5
  Constant45/1 -> A8/4
  Constant85/1 -> A8/2
  Constant49/1 -> A8/8
  Constant52/1 -> A9/4
  Constant56/1 -> A9/7
  Constant51/1 -> A9/3
  Constant57/1 -> A9/8
  Constant44/1 -> A8/3
  Constant46/1 -> A8/5
  Constant50/1 -> A9/2
  Constant48/1 -> A8/7
  Constant60/1 -> A10/4
  Constant62/1 -> A10/6
  Constant63/1 -> A10/7
  Constant64/1 -> A10/8
  Constant67/1 -> A11/3
  Constant66/1 -> A11/2
  Constant84/1 -> A7/8
  Constant59/1 -> A10/3
  Constant58/1 -> A10/2
  A9/1 -> Out3/1
  A8/1 -> Out2/1
  Constant65/1 -> A7/3
  A12/1 -> Out6/1
  A11/1 -> Out5/1
  A7/1 -> Out1/1
  Constant54/1 -> A7/2
  Constant76/1 -> A7/4
  A10/1 -> Out4/1
  Constant81/1 -> A7/5
  Constant82/1 -> A7/6
  Constant83/1 -> A7/7

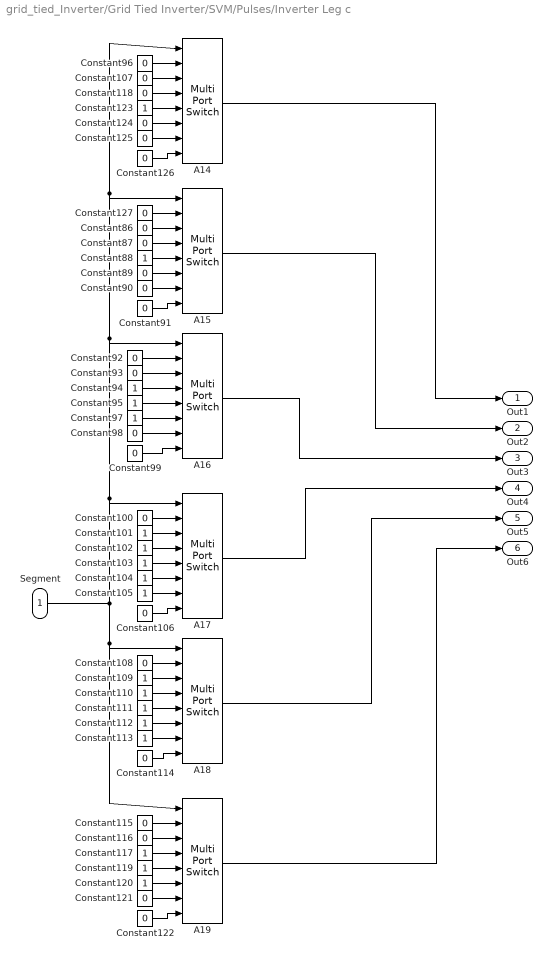
== system grid_tied_Inverter/Grid Tied Inverter/SVM/Pulses/Inverter Leg c ==
  Segment : Inport
  A{14..19} (6 alike) : MultiPortSwitch  Inputs=7
  Constant{86..87,89..93,96,98..100,106..108,114..116,118,121..122,124..127} (24 alike) : Constant  Value=0
  Constant{88,94..95,97,101..105,109..113,117,119..120,123} (18 alike) : Constant
  Out1 : Outport
  Out2 : Outport  Port=2
  Out3 : Outport  Port=3
  Out4 : Outport  Port=4
  Out5 : Outport  Port=5
  Out6 : Outport  Port=6
  wires:
  Constant86/1 -> A15/3
  Constant103/1 -> A17/5
  Constant88/1 -> A15/5
  Constant101/1 -> A17/3
  Constant127/1 -> A15/2
  Constant102/1 -> A17/4
  Constant104/1 -> A17/6
  Constant100/1 -> A17/2
  Constant97/1 -> A16/6
  Constant94/1 -> A16/4
  Constant99/1 -> A16/8
  Constant105/1 -> A17/7
  Constant110/1 -> A18/4
  Constant109/1 -> A18/3
  Constant89/1 -> A15/6
  Constant113/1 -> A18/7
  Constant114/1 -> A18/8
  Constant87/1 -> A15/4
  Constant98/1 -> A16/7
  Constant91/1 -> A15/8
  Constant108/1 -> A18/2
  Constant92/1 -> A16/2
  Constant116/1 -> A19/3
  Constant111/1 -> A18/5
  Constant115/1 -> A19/2
  Constant117/1 -> A19/4
  Constant119/1 -> A19/5
  Constant112/1 -> A18/6
  Constant93/1 -> A16/3
  Constant95/1 -> A16/5
  Constant90/1 -> A15/7
  Constant106/1 -> A17/8
  Constant122/1 -> A19/8
  Constant121/1 -> A19/7
  Constant120/1 -> A19/6
  Segment/1 -> A15/1, A14/1, A16/1, A17/1, A19/1, A18/1
  Constant126/1 -> A14/8
  A16/1 -> Out3/1
  A17/1 -> Out4/1
  Constant96/1 -> A14/2
  Constant118/1 -> A14/4
  A18/1 -> Out5/1
  Constant107/1 -> A14/3
  A19/1 -> Out6/1
  Constant123/1 -> A14/5
  A15/1 -> Out2/1
  Constant124/1 -> A14/6
  A14/1 -> Out1/1
  Constant125/1 -> A14/7

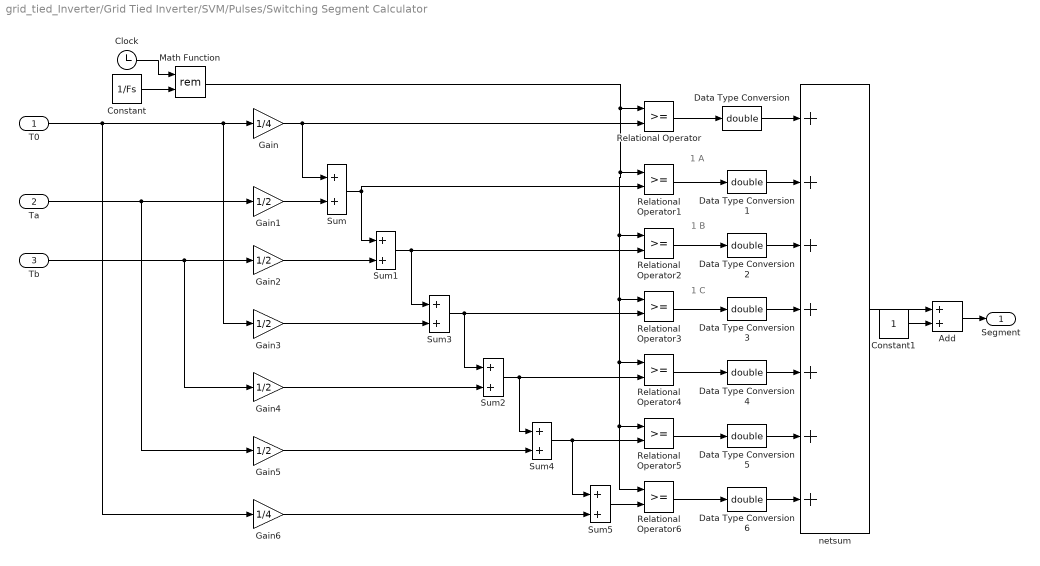
== system grid_tied_Inverter/Grid Tied Inverter/SVM/Pulses/Switching Segment Calculator ==
  note: 1 A
  note: 1 B
  note: 1 C
  T0 : Inport
  Ta : Inport  Port=2
  Tb : Inport  Port=3
  Add : Sum
  Clock : Clock
  Constant : Constant  Value=1/Fs
  Constant1 : Constant
  Data Type Conversion{,1..6} (7 alike) : DataTypeConversion  OutDataTypeStr=double
  Gain : Gain  Gain=1/4
  Gain{1..5} (5 alike) : Gain  Gain=1/2
  Gain6 : Gain  Gain=1/4
  Math Function : Math  Operator=rem  SaturateOnIntegerOverflow=on
  Relational Operator{,1..6} (7 alike) : RelationalOperator  OutDataTypeStr=boolean
  Sum{,1..5} (6 alike) : Sum
  netsum : Sum  Inputs=7  SaturateOnIntegerOverflow=on  InputSameDT=on  OutDataTypeStr=Inherit: Same as first input
  Segment : Outport
  wires:
  Ta/1 -> Gain5/1, Gain1/1
  Gain2/1 -> Sum1/2
  Sum4/1 -> Sum5/1, Relational Operator5/2
  Math Function/1 -> Relational Operator6/1, Relational Operator5/1, Relational Operator4/1, Relational Operator3/1, Relational Operator2/1, Relational Operator1/1, Relational Operator/1
  Gain4/1 -> Sum2/2
  Gain5/1 -> Sum4/2
  Relational Operator/1 -> Data Type Conversion/1
  Relational Operator1/1 -> Data Type Conversion1/1
  Relational Operator2/1 -> Data Type Conversion2/1
  Sum3/1 -> Sum2/1, Relational Operator3/2
  Constant/1 -> Math Function/2
  Relational Operator3/1 -> Data Type Conversion3/1
  Gain3/1 -> Sum3/2
  Sum5/1 -> Relational Operator6/2
  Sum1/1 -> Sum3/1, Relational Operator2/2
  Gain6/1 -> Sum5/2
  Clock/1 -> Math Function/1
  Tb/1 -> Gain4/1, Gain2/1
  Sum/1 -> Sum1/1, Relational Operator1/2
  Gain/1 -> Sum/1, Relational Operator/2
  Gain1/1 -> Sum/2
  Sum2/1 -> Sum4/1, Relational Operator4/2
  Data Type Conversion3/1 -> netsum/4
  netsum/1 -> Add/1
  Data Type Conversion2/1 -> netsum/3
  Constant1/1 -> Add/2
  Data Type Conversion1/1 -> netsum/2
  Relational Operator4/1 -> Data Type Conversion4/1
  Data Type Conversion4/1 -> netsum/5
  Data Type Conversion6/1 -> netsum/7
  Data Type Conversion/1 -> netsum/1
  Relational Operator6/1 -> Data Type Conversion6/1
  Data Type Conversion5/1 -> netsum/6
  Relational Operator5/1 -> Data Type Conversion5/1
  Add/1 -> Segment/1
  T0/1 -> Gain6/1, Gain3/1, Gain/1
